simulink model "MIAC_ZTransform_PLC_Coder_not_external"  (R2018b)
settings: Solver=FixedStepDiscrete  StartTime=0.0  StopTime=20  FixedStep=1  RelTol=1e-3
libraries: simulink x2, slident x2
settings Model: Creator=Trips  LastModifiedBy=Trips
settings ConfigComp: PLC_OutputDir=PLCCoder  PLC_TargetIDE=step7  PLC_GenerateReport=off  PLC_LaunchReport=off

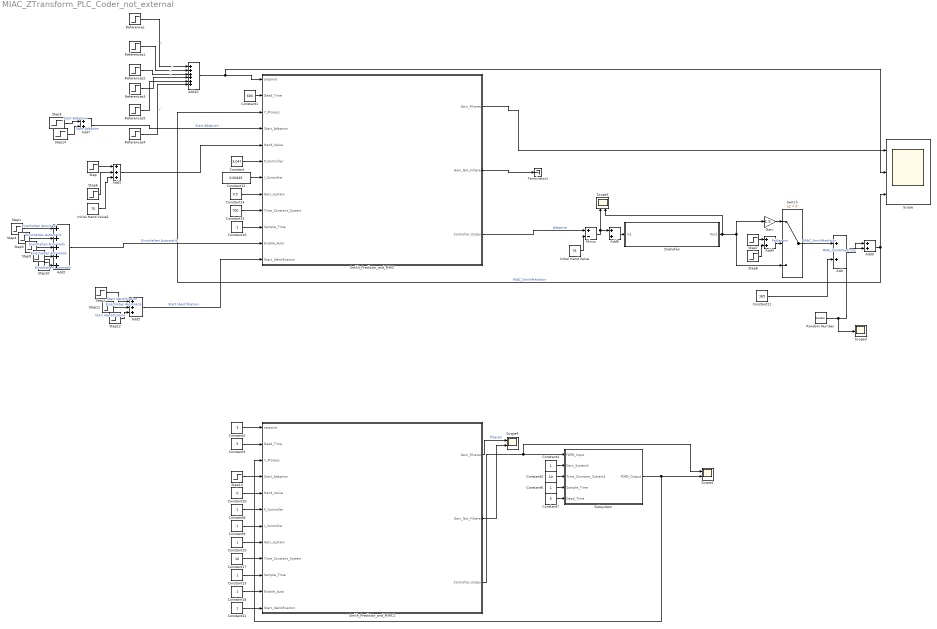
== system MIAC_ZTransform_PLC_Coder_not_external ==
  Add{,3..4,6..7} (5 alike) : Sum
  Add1 : Sum  Inputs=+++
  Add10 : Sum  Inputs=++++++
  Add2 : Sum  Inputs=5
  Add5 : Sum  Inputs=+++
  Constant : Constant  Value=3.047
  Constant1 : Constant  Value=600
  Constant{4,6,8..10,13,16,18,21} (9 alike) : Constant
  Constant11 : Constant  Value=165
  Constant12 : Constant  Value=0.00445
  Constant14 : Constant  Value=0.5
  Constant15 : Constant  Value=700
  Constant17 : Constant  Value=10
  Constant2 : Constant  Value=3
  Constant20 : Constant  Value=0
  Constant3 : Constant  Value=5
  Constant5 : Constant  Value=10
  Constant7 : Constant  Value=5
  Drehofen : Subsystem
  Gain : Gain  Gain=1.5
  Initial Hand Value : Constant  Value=75
  Initial Hand Value1 : Constant  Value=75
  Minus : Sum  Inputs=+-
  Random Number : RandomNumber  Variance=0.01  SampleTime=10
  References : Step  After=3
  References1 : Step  Time=12000  After=2
  References2 : Step  Time=18000  After=3
  References3 : Step  Time=35000  After=3
  References4 : Step  Time=0  After=165
  References5 : Step  Time=40000  After=-7
  Scope : Scope  NumInputPorts=3
  Scope1 : Scope  NumInputPorts=2
  Scope2 : Scope  NumInputPorts=2
  Scope3 : Scope
  Scope4 : Scope  NumInputPorts=2
  Smith_Predictor_and_MIAC : Subsystem  TreatAsAtomicUnit=on  SystemSampleTime=1
  Smith_Predictor_and_MIAC1 : Subsystem  TreatAsAtomicUnit=on  SystemSampleTime=1
  Step : Step  Time=300  After=5  SampleTime=0
  Step1 : Step  Time=4000  SampleTime=0
  Step10 : Step  Time=50000  SampleTime=0
  Step11 : Step  Time=35000  After=-1  SampleTime=0
  Step12 : Step  Time=38000  SampleTime=1
  Step13 : Step  Time=500  SampleTime=0
  Step14 : Step  Time=2.5*10^4  SampleTime=1
  Step2 : Step  Time=3900  SampleTime=1
  Step3 : Step  Time=5000  Before=1  After=0  SampleTime=1
  Step4 : Step  Time=20000  After=-1  SampleTime=0
  Step5 : Step  Time=25000  SampleTime=0
  Step6 : Step  Time=19000  After=5  SampleTime=0
  Step7 : Step  Time=3*10^4  SampleTime=0
  Step8 : Step  Time=3.8*10^4  After=0  SampleTime=0
  Step9 : Step  Time=45000  After=-1  SampleTime=0
  Subsystem : Subsystem  TreatAsAtomicUnit=on  SystemSampleTime=1
  Switch : Switch  Criteria=u2 > Threshold
  Terminator1 : Terminator
  wires:
  Smith_Predictor_and_MIAC/1(Gain_Filtered) -> Scope/1
  Smith_Predictor_and_MIAC/2(Gain_Not_Filtered) -> Terminator1/1
  Add10/1 -> Scope/2, Smith_Predictor_and_MIAC/1(setpoint)
  Step8/1 -> Add4/2
  Smith_Predictor_and_MIAC/3(Controller_Output) -> Minus/1  "Adaptive"
  Add4/1 -> Switch/2  "Fehler ein"
  Gain/1 -> Switch/1
  Minus/1 -> Add6/1, Scope1/1
  Add6/1 -> Drehofen/1(In1)
  Drehofen/1(Out1) -> Scope1/2, Gain/1, Switch/3
  Step7/1 -> Add4/1
  Random Number/1 -> Scope3/1, Add3/2
  Initial Hand Value/1 -> Minus/2
  Add/1 -> Add3/1  "MIAC_SmithPredictor"
  Switch/1 -> Add/1  "MIAC_SmithPredictor"
  Constant11/1 -> Add/2
  Add3/1 -> Scope/3, Smith_Predictor_and_MIAC/3(Y_Process)  "MIAC_SmithPredictor"
  References3/1 -> Add10/4  "r"
  References/1 -> Add10/1  "r"
  References4/1 -> Add10/6  "r"
  References1/1 -> Add10/2  "r"
  References2/1 -> Add10/3  "r"
  References5/1 -> Add10/5
  Constant/1 -> Smith_Predictor_and_MIAC/6(P_Controller)
  Constant12/1 -> Smith_Predictor_and_MIAC/7(I_Controller)
  Constant14/1 -> Smith_Predictor_and_MIAC/8(Gain_System)
  Constant15/1 -> Smith_Predictor_and_MIAC/9(Time_Constant_System)
  Constant16/1 -> Smith_Predictor_and_MIAC/10(Sample_Time)
  Constant1/1 -> Smith_Predictor_and_MIAC/2(Dead_Time)
  Step14/1 -> Add7/2  "Start Adaption"
  Step3/1 -> Add7/1  "Start Adaption"
  Add7/1 -> Smith_Predictor_and_MIAC/4(Start_Adaption)  "Start Adaption"
  Step6/1 -> Add1/2
  Initial Hand Value1/1 -> Add1/3
  Step/1 -> Add1/1
  Add1/1 -> Smith_Predictor_and_MIAC/5(Hand_Value)
  Step9/1 -> Add2/4  "Einschalten Automatik"
  Step10/1 -> Add2/5  "Einschalten Automatik"
  Step5/1 -> Add2/3  "Einschalten Automatik"
  Step4/1 -> Add2/2  "Einschalten Automatik"
  Step1/1 -> Add2/1  "Einschalten Automatik"
  Add2/1 -> Smith_Predictor_and_MIAC/11(" Enable_Auto")  "Einschalten Automatik"
  Step12/1 -> Add5/3  "Start Identification"
  Step11/1 -> Add5/2  "Einschalten Automatik"
  Step2/1 -> Add5/1  "Start Identification"
  Add5/1 -> Smith_Predictor_and_MIAC/12(Start_Identification)  "Start Identification"
  Constant2/1 -> Smith_Predictor_and_MIAC1/1(setpoint)
  Constant3/1 -> Smith_Predictor_and_MIAC1/2(Dead_Time)
  Constant7/1 -> Subsystem/5(" Dead_Time")
  Constant4/1 -> Subsystem/2(Gain_System1)
  Constant6/1 -> Subsystem/4(Sample_Time)
  Subsystem/1(FOPD_Output) -> Smith_Predictor_and_MIAC1/3(Y_Process), Scope2/2
  Constant5/1 -> Subsystem/3(Time_Constant_System1)
  Smith_Predictor_and_MIAC1/3(Controller_Output) -> Scope2/1, Subsystem/1(FOPD_Input)
  Constant8/1 -> Smith_Predictor_and_MIAC1/6(P_Controller)
  Constant9/1 -> Smith_Predictor_and_MIAC1/7(I_Controller)
  Constant10/1 -> Smith_Predictor_and_MIAC1/8(Gain_System)
  Constant13/1 -> Smith_Predictor_and_MIAC1/10(Sample_Time)
  Constant17/1 -> Smith_Predictor_and_MIAC1/9(Time_Constant_System)
  Constant18/1 -> Smith_Predictor_and_MIAC1/11(" Enable_Auto")
  Step13/1 -> Smith_Predictor_and_MIAC1/4(Start_Adaption)
  Constant20/1 -> Smith_Predictor_and_MIAC1/5(Hand_Value)
  Constant21/1 -> Smith_Predictor_and_MIAC1/12(Start_Identification)
  Smith_Predictor_and_MIAC1/1(Gain_Filtered) -> Scope4/1  "filtered"
  Smith_Predictor_and_MIAC1/2(Gain_Not_Filtered) -> Scope4/2

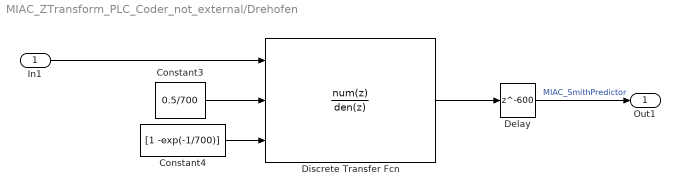
== system MIAC_ZTransform_PLC_Coder_not_external/Drehofen ==
  In1 : Inport
  Constant3 : Constant  Value=0.5/700
  Constant4 : Constant  Value=[1 -exp(-1/700)]
  Delay : Delay  DelayLength=600
  Discrete Transfer Fcn : DiscreteTransferFcn  NumeratorSource=Input port  DenominatorSource=Input port  a0EqualsOne=on
      settings: InputPortMap=u0,p1,p3
  Out1 : Outport
  wires:
  Discrete Transfer Fcn/1 -> Delay/1
  Constant4/1 -> Discrete Transfer Fcn/3
  Constant3/1 -> Discrete Transfer Fcn/2
  In1/1 -> Discrete Transfer Fcn/1
  Delay/1 -> Out1/1  "MIAC_SmithPredictor"

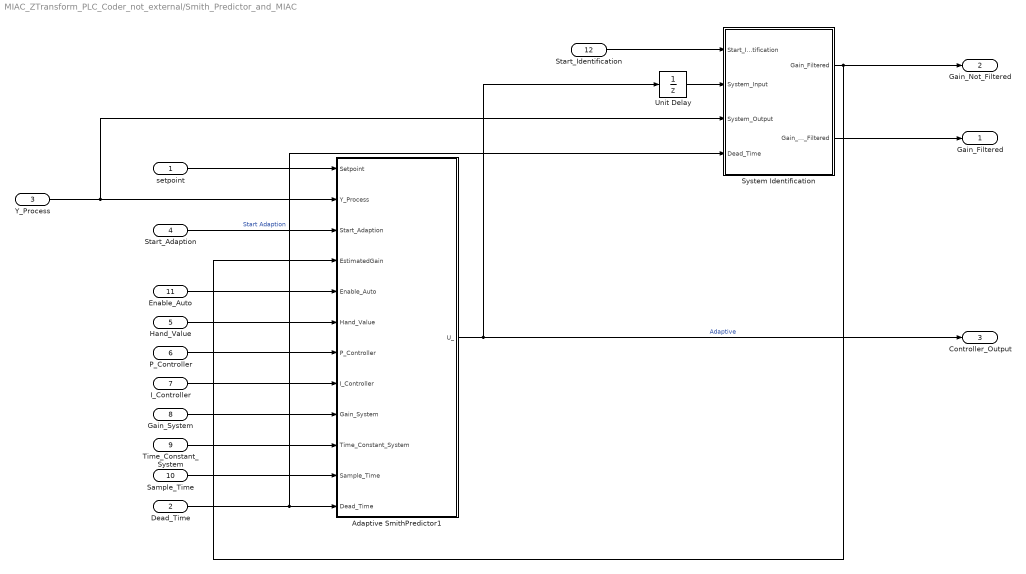
== system MIAC_ZTransform_PLC_Coder_not_external/Smith_Predictor_and_MIAC ==
  setpoint : Inport
  Dead_Time : Inport  Port=2
  Y_Process : Inport  Port=3
  Start_Adaption : Inport  Port=4
  Hand_Value : Inport  Port=5
  P_Controller : Inport  Port=6
  I_Controller : Inport  Port=7
  Gain_System : Inport  Port=8
  Time_Constant_System : Inport  Port=9
  Sample_Time : Inport  Port=10
  " Enable_Auto" : Inport  Port=11
  Start_Identification : Inport  Port=12  PortDimensions=1  SampleTime=1
  Adaptive SmithPredictor1 : Subsystem  TreatAsAtomicUnit=on  SystemSampleTime=1
  System Identification : Subsystem  TreatAsAtomicUnit=on  SystemSampleTime=1
  Unit Delay : UnitDelay  SampleTime=-1
  Gain_Filtered : Outport
  Gain_Not_Filtered : Outport  Port=2
  Controller_Output : Outport  Port=3
  wires:
  Gain_System/1 -> Adaptive SmithPredictor1/9(Gain_System)
  Dead_Time/1 -> Adaptive SmithPredictor1/12(" Dead_Time"), System Identification/4(Dead_Time)
  Adaptive SmithPredictor1/1(U_) -> Unit Delay/1, Controller_Output/1  "Adaptive"
  Time_Constant_System/1 -> Adaptive SmithPredictor1/10(Time_Constant_System)
  P_Controller/1 -> Adaptive SmithPredictor1/7(P_Controller)
  Sample_Time/1 -> Adaptive SmithPredictor1/11(Sample_Time)
  I_Controller/1 -> Adaptive SmithPredictor1/8(I_Controller)
  Start_Adaption/1 -> Adaptive SmithPredictor1/3(Start_Adaption)  "Start Adaption"
  System Identification/2(Gain_Not_Filtered) -> Gain_Filtered/1
  setpoint/1 -> Adaptive SmithPredictor1/1(Setpoint)
  Start_Identification/1 -> System Identification/1(Start_Identification)
  System Identification/1(Gain_Filtered) -> Adaptive SmithPredictor1/4(EstimatedGain), Gain_Not_Filtered/1
  " Enable_Auto"/1 -> Adaptive SmithPredictor1/5(Enable_Auto)
  Hand_Value/1 -> Adaptive SmithPredictor1/6(Hand_Value)
  Y_Process/1 -> System Identification/3(System_Output), Adaptive SmithPredictor1/2(Y_Process)
  Unit Delay/1 -> System Identification/2(System_Input)

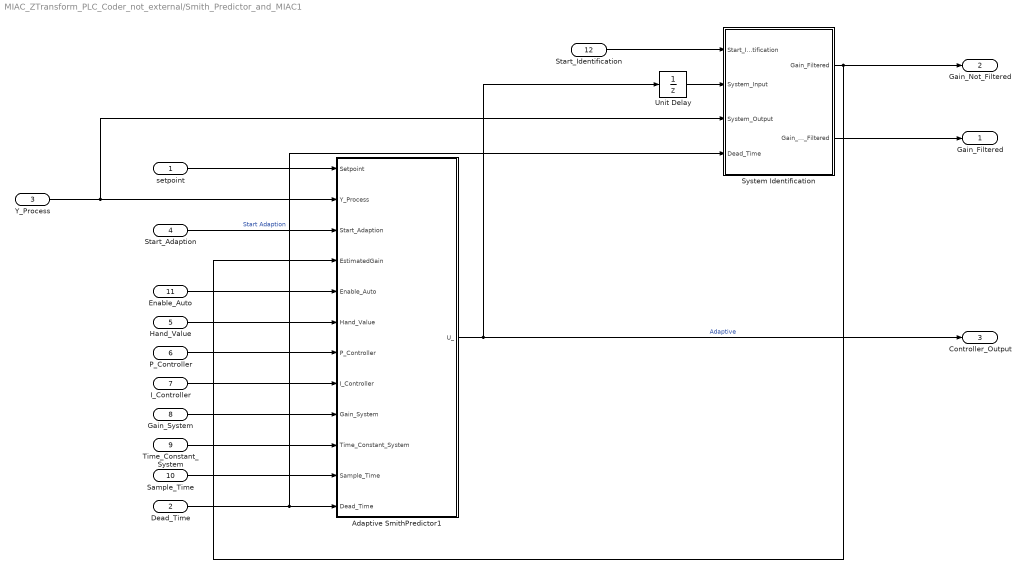
== system MIAC_ZTransform_PLC_Coder_not_external/Smith_Predictor_and_MIAC1 ==
  setpoint : Inport
  Dead_Time : Inport  Port=2
  Y_Process : Inport  Port=3
  Start_Adaption : Inport  Port=4
  Hand_Value : Inport  Port=5
  P_Controller : Inport  Port=6
  I_Controller : Inport  Port=7
  Gain_System : Inport  Port=8
  Time_Constant_System : Inport  Port=9
  Sample_Time : Inport  Port=10
  " Enable_Auto" : Inport  Port=11
  Start_Identification : Inport  Port=12  PortDimensions=1  SampleTime=1
  Adaptive SmithPredictor1 : Subsystem  TreatAsAtomicUnit=on  SystemSampleTime=1
  System Identification : Subsystem  TreatAsAtomicUnit=on  SystemSampleTime=1
  Unit Delay : UnitDelay  SampleTime=-1
  Gain_Filtered : Outport
  Gain_Not_Filtered : Outport  Port=2
  Controller_Output : Outport  Port=3
  wires:
  Gain_System/1 -> Adaptive SmithPredictor1/9(Gain_System)
  Dead_Time/1 -> Adaptive SmithPredictor1/12(" Dead_Time"), System Identification/4(Dead_Time)
  Adaptive SmithPredictor1/1(U_) -> Unit Delay/1, Controller_Output/1  "Adaptive"
  Time_Constant_System/1 -> Adaptive SmithPredictor1/10(Time_Constant_System)
  P_Controller/1 -> Adaptive SmithPredictor1/7(P_Controller)
  Sample_Time/1 -> Adaptive SmithPredictor1/11(Sample_Time)
  I_Controller/1 -> Adaptive SmithPredictor1/8(I_Controller)
  Start_Adaption/1 -> Adaptive SmithPredictor1/3(Start_Adaption)  "Start Adaption"
  System Identification/2(Gain_Not_Filtered) -> Gain_Filtered/1
  setpoint/1 -> Adaptive SmithPredictor1/1(Setpoint)
  Start_Identification/1 -> System Identification/1(Start_Identification)
  System Identification/1(Gain_Filtered) -> Adaptive SmithPredictor1/4(EstimatedGain), Gain_Not_Filtered/1
  " Enable_Auto"/1 -> Adaptive SmithPredictor1/5(Enable_Auto)
  Hand_Value/1 -> Adaptive SmithPredictor1/6(Hand_Value)
  Y_Process/1 -> System Identification/3(System_Output), Adaptive SmithPredictor1/2(Y_Process)
  Unit Delay/1 -> System Identification/2(System_Input)

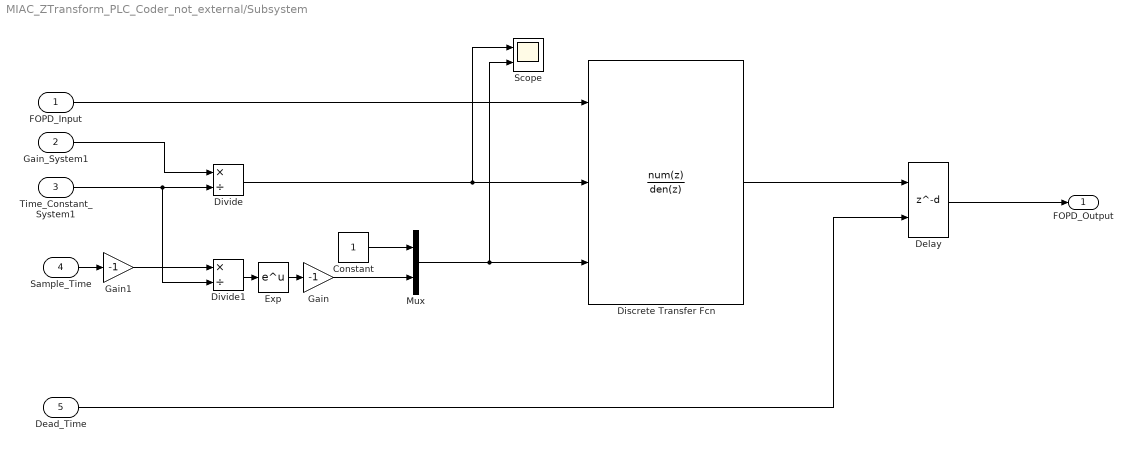
== system MIAC_ZTransform_PLC_Coder_not_external/Subsystem ==
  FOPD_Input : Inport
  Gain_System1 : Inport  Port=2
  Time_Constant_System1 : Inport  Port=3
  Sample_Time : Inport  Port=4
  " Dead_Time" : Inport  Port=5
  Constant : Constant
  Delay : Delay  DelayLengthSource=Input port  DelayLength=600  DelayLengthUpperLimit=800
      settings: InputPortMap=u0,p1
  Discrete Transfer Fcn : DiscreteTransferFcn  NumeratorSource=Input port  DenominatorSource=Input port  a0EqualsOne=on
      settings: InputPortMap=u0,p1,p3
  Divide : Product  Inputs=*/
  Divide1 : Product  Inputs=*/
  Exp : Math  SaturateOnIntegerOverflow=on
  Gain : Gain  Gain=-1
  Gain1 : Gain  Gain=-1
  Mux : Mux  Inputs=2
  Scope : Scope  NumInputPorts=2
  FOPD_Output : Outport
  wires:
  Gain1/1 -> Divide1/1
  Time_Constant_System1/1 -> Divide1/2, Divide/2
  FOPD_Input/1 -> Discrete Transfer Fcn/1
  Discrete Transfer Fcn/1 -> Delay/1
  Exp/1 -> Gain/1
  Constant/1 -> Mux/1
  Mux/1 -> Scope/2, Discrete Transfer Fcn/3
  Divide1/1 -> Exp/1
  Gain_System1/1 -> Divide/1
  Gain/1 -> Mux/2
  " Dead_Time"/1 -> Delay/2
  Sample_Time/1 -> Gain1/1
  Divide/1 -> Scope/1, Discrete Transfer Fcn/2
  Delay/1 -> FOPD_Output/1

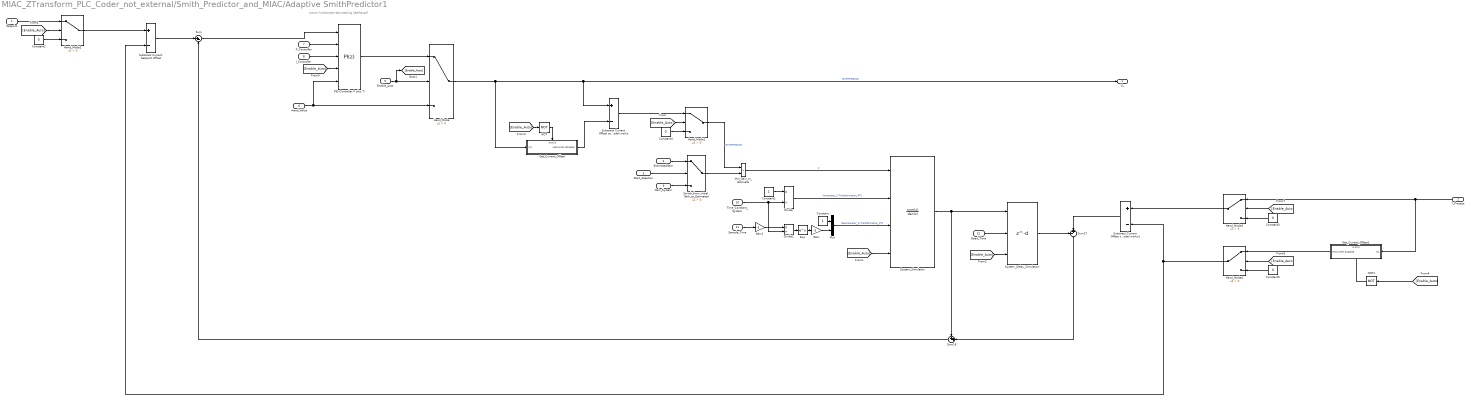
== system MIAC_ZTransform_PLC_Coder_not_external/Smith_Predictor_and_MIAC/Adaptive SmithPredictor1 ==
  note: warum funktioniert das tracking überhaupt?
  Setpoint : Inport
  Y_Process : Inport  Port=2
  Start_Adaption : Inport  Port=3
  EstimatedGain : Inport  Port=4
  Enable_Auto : Inport  Port=5
  Hand_Value : Inport  Port=6
  P_Controller : Inport  Port=7
  I_Controller : Inport  Port=8
  Gain_System : Inport  Port=9
  Time_Constant_System : Inport  Port=10
  Sample_Time : Inport  Port=11
  " Dead_Time" : Inport  Port=12
  Constant : Constant
  Constant1 : Constant
  Constant{2..5} (4 alike) : Constant  Value=0
  Divide : Product  Inputs=*/
  Divide1 : Product  Inputs=*/
  Exp : Math  SaturateOnIntegerOverflow=on
  Gain : Gain  Gain=-1
  Gain1 : Gain  Gain=-1
  Get_Current_Offset : Subsystem
  Get_Current_Offset1 : Subsystem
  Hand_Mode{,1..4} (5 alike) : Switch  Criteria=u2 > Threshold
  Mul_Gain_or_Estimate : Product
  Mux : Mux  Inputs=2
  NOT : Logic  Operator=NOT  IconShape=distinctive  AllPortsSameDT=off  OutDataTypeStr=boolean
  NOT1 : Logic  Operator=NOT  IconShape=distinctive  AllPortsSameDT=off  OutDataTypeStr=boolean
  "PID Controller P plus Ti " : simulink/Continuous/PID Controller  Controller=PI  Form=Parallel  TimeDomain=Discrete-time  SampleTime=1  IntegratorMethod=Forward Euler  FilterMethod=Forward Euler  ControllerParametersSource=external  P=3.04732259067536  I=0.00445689106465138  D=118.272348286844  UseFilter=on  N=0.00420306193364532  TunerSelectOption=Transfer Function Based (PID Tuner App)  InitialConditionSource=external  InitialConditionForIntegrator=0  InitialConditionForFilter=0  DifferentiatorICPrevScaledInput=0  ExternalReset=rising  TrackingMode=off  Kt=1  LimitOutput=on  UpperSaturationLimit=100  LowerSaturationLimit=0  LinearizeAsGain=on  AntiWindupMode=none  Kb=1  POutMin=[]  POutMax=[]  IOutMin=[]  IOutMax=[]  DOutMin=[]  DOutMax=[]  NOutMin=[]  NOutMax=[]  SumOutMin=[]  SumOutMax=[]  SaturationOutMin=[]  SaturationOutMax=[]  PParamMin=[]  PParamMax=[]  IParamMin=[]  IParamMax=[]  DParamMin=[]  DParamMax=[]  NParamMin=[]  NParamMax=[]  KbParamMin=[]  KbParamMax=[]  KtParamMin=[]  KtParamMax=[]  KbOutMin=[]  KbOutMax=[]  KtOutMin=[]  KtOutMax=[]  IntegratorOutMin=[]  IntegratorOutMax=[]  FilterOutMin=[]  FilterOutMax=[]  SumI1OutMin=[]  SumI1OutMax=[]  SumI2OutMin=[]  SumI2OutMax=[]  SumI3OutMin=[]  SumI3OutMax=[]  SumI4OutMin=[]  SumI4OutMax=[]  SumDOutMin=[]  SumDOutMax=[]  DifferentiatorOutMin=[]  DifferentiatorOutMax=[]  FilterDiffOutCoefMin=[]  FilterDiffOutCoefMax=[]  ReciprocalOutMin=[]  ReciprocalOutMax=[]  SumDenOutMin=[]  SumDenOutMax=[]  SumNumOutMin=[]  SumNumOutMax=[]  DivideOutMin=[]  DivideOutMax=[]  IntegratorContinuousStateAttributes=''  IntegratorStateMustResolveToSignalObject=off  IntegratorRTWStateStorageClass=Auto  FilterContinuousStateAttributes=''  FilterStateMustResolveToSignalObject=off  FilterRTWStateStorageClass=Auto  ParallelPVariant=ExternalParameters  IdealPVariant=Disabled  IVariant=ExternalParameters  DVariant=Disabled  IntegratorVariant=Discrete  SatVariant=Enabled  AWVariant=Passthrough  PCopyVariant=Disabled  TRVariant=Disabled  FdbkBlocksVariant=Forward  IdealPFdbkVariant=Disabled  SatFdbkVariant=Disabled  DerivativeFilterVariant=Disabled  NVariant=Disabled  NCopyVariant=Disabled_SignalSpec  FilterICVariant=Disabled  IntegratorICVariant=ExternalICs  ExternalResetVariant=ExternalReset  TRSumVariant=Passthrough  SumFdbkVariant=Disabled  SumVariant=Sum_PI
  Substract Current Offset so that the linearised model works : Sum  Inputs=+-
  Substract Current Offset so that the linearised model works1 : Sum  Inputs=+-
  Substract Current Setpoint Offset : Sum  Inputs=+-
  Sum : Sum  Inputs=|+-
  Sum17 : Sum  Inputs=-+|
  Sum18 : Sum  Inputs=++|
  Switch_from_initial_Gain_to_Estimated : Switch  Criteria=u2 > Threshold
  System_Delay_Simulation : Delay  DelayLengthSource=Input port  DelayLength=600  DelayLengthUpperLimit=800  ExternalReset=Rising  SampleTime=1
      settings: InputPortMap=u0,p1,r5
  System_Simulaton : DiscreteTransferFcn  NumeratorSource=Input port  DenominatorSource=Input port  ExternalReset=Rising  SampleTime=1  a0EqualsOne=on
      settings: InputPortMap=u0,p1,p3,r7
  U_ : Outport
  wires:
  Substract Current Setpoint Offset/1 -> Sum/1
  Sum/1 -> "PID Controller P plus Ti "/1
  Hand_Mode/1 -> U_/1, Substract Current Offset so that the linearised model works/1, Get_Current_Offset/1(In1)  "SmithPredictor"
  Substract Current Offset so that the linearised model works1/1 -> Sum17/2
  System_Simulaton/1 -> Sum18/1, System_Delay_Simulation/1
  System_Delay_Simulation/1 -> Sum17/1
  Sum17/1 -> Sum18/2
  Mul_Gain_or_Estimate/1 -> System_Simulaton/1  "U"
  Switch_from_initial_Gain_to_Estimated/1 -> Mul_Gain_or_Estimate/2
  "PID Controller P plus Ti "/1 -> Hand_Mode/1
  Hand_Value/1 -> "PID Controller P plus Ti "/5, Hand_Mode/3
  Enable_Auto/1 -> [Enable_Auto], Hand_Mode/2
  P_Controller/1 -> "PID Controller P plus Ti "/2
  I_Controller/1 -> "PID Controller P plus Ti "/3
  Divide/1 -> System_Simulaton/2  "Numerator_Z-Transformation_PT1"
  Mux/1 -> System_Simulaton/3  "Denumerator_Z-Transformation_PT1"
  Time_Constant_System/1 -> Divide1/2, Divide/2
  Constant/1 -> Mux/1
  Exp/1 -> Gain/1
  Gain/1 -> Mux/2
  Divide1/1 -> Exp/1
  Sample_Time/1 -> Gain1/1
  " Dead_Time"/1 -> System_Delay_Simulation/2
  Gain_System/1 -> Switch_from_initial_Gain_to_Estimated/3
  Start_Adaption/1 -> Switch_from_initial_Gain_to_Estimated/2
  EstimatedGain/1 -> Switch_from_initial_Gain_to_Estimated/1
  Constant1/1 -> Divide/1
  Gain1/1 -> Divide1/1
  [Enable_Auto] -> Hand_Mode1/2
  Hand_Mode1/1 -> Mul_Gain_or_Estimate/1  "SmithPredictor"
  Constant4/1 -> Hand_Mode1/3
  [Enable_Auto] -> System_Simulaton/4
  [Enable_Auto] -> System_Delay_Simulation/3
  Substract Current Offset so that the linearised model works/1 -> Hand_Mode1/1
  Get_Current_Offset/1(Hold when disabled) -> Substract Current Offset so that the linearised model works/2
  [Enable_Auto] -> NOT/1
  NOT/1 -> Get_Current_Offset/Enable
  Sum18/1 -> Sum/2
  Hand_Mode2/1 -> Substract Current Setpoint Offset/1
  NOT1/1 -> Get_Current_Offset1/Enable
  [Enable_Auto] -> NOT1/1
  Hand_Mode4/1 -> Substract Current Setpoint Offset/2, Substract Current Offset so that the linearised model works1/2
  [Enable_Auto] -> "PID Controller P plus Ti "/4
  Setpoint/1 -> Hand_Mode2/1
  [Enable_Auto] -> Hand_Mode2/2
  Constant2/1 -> Hand_Mode2/3
  Y_Process/1 -> Get_Current_Offset1/1(In1), Hand_Mode3/1
  [Enable_Auto] -> Hand_Mode3/2
  Constant3/1 -> Hand_Mode3/3
  Hand_Mode3/1 -> Substract Current Offset so that the linearised model works1/1
  Constant5/1 -> Hand_Mode4/3
  [Enable_Auto] -> Hand_Mode4/2
  Get_Current_Offset1/1(Hold when disabled) -> Hand_Mode4/1

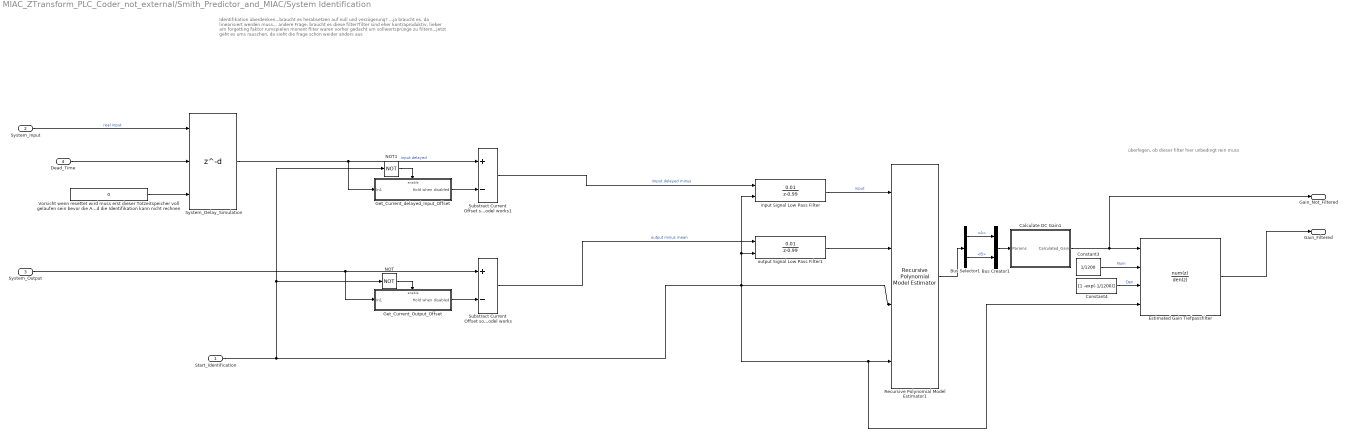
== system MIAC_ZTransform_PLC_Coder_not_external/Smith_Predictor_and_MIAC/System Identification ==
  note: überlegen, ob dieser filter hier unbedingt rein muss
  note: Identifikation überdenken...braucht es herabsetzen auf null und verzögerung?
      | ...ja braucht es, da linearisiert werden muss...
      |
      | andere Frage, braucht es diese filter?filter sind eher kontraproduktiv, lieber am forgetting faktor rumspielen
      | monent fliter waren vorher gedacht um sollwertsprünge zu filtern...jetzt geht es ums rauschen, da sieht die frage schon weider anders aus
  Start_Identification : Inport  SampleTime=1
  System_Input : Inport  Port=2
  System_Output : Inport  Port=3  SampleTime=1
  Dead_Time : Inport  Port=4
  Bus Creator1 : BusCreator  Inputs=2
  Bus Selector1 : BusSelector  OutputSignals=A,B
  Calculate DC Gain1 : Subsystem  TreatAsAtomicUnit=on  SystemSampleTime=1
  Constant3 : Constant  Value=1/1200
  Constant4 : Constant  Value=[1 -exp(-1/1200)]
  Estimated Gain Tiefpassfilter : DiscreteTransferFcn  NumeratorSource=Input port  DenominatorSource=Input port  ExternalReset=Rising  a0EqualsOne=on
      settings: InputPortMap=u0,p1,p3,r7
  Get_Current_Output_Offset : Subsystem
  Get_Current_delayed_Input_Offset : Subsystem
  NOT : Logic  Operator=NOT  IconShape=distinctive  AllPortsSameDT=off  OutDataTypeStr=boolean
  NOT1 : Logic  Operator=NOT  IconShape=distinctive  AllPortsSameDT=off  OutDataTypeStr=boolean
  Recursive Polynomial Model Estimator1 : slident/Estimators/Recursive Polynomial Model Estimator  ModelStructure=ARX  InitialEstimateSource=None  A0=2  B0=1  C0=1  D0=1  F0=1  nk=1  P0=10  InitialInputs=0  InitialOutputs=0  History=Infinite  WindowLength=2000  EstimationMethod=Forgetting Factor  AdaptationParameter=1  HasTimeVaryingAdaptationParameter=off  NormalizationBias=eps  OutputError=off  OutputP=off  AddEnablePort=on  ExternalReset=Rising  InputProcessing=Sample-based  Ts=1
      settings: SourceProductName=System Identification Toolbox  SourceProductBaseCode=ID
  Substract Current Offset so that the linearised model works : Sum  Inputs=+-
  Substract Current Offset so that the linearised model works1 : Sum  Inputs=+-
  System_Delay_Simulation : Delay  DelayLengthSource=Input port  DelayLength=600  DelayLengthUpperLimit=800  ExternalReset=Rising  SampleTime=1
      settings: InputPortMap=u0,p1,r5
  Vorsicht wenn resettet wird muss erst dieser Totzeitspeicher voll gelaufen sein bevor die Adaption starten darf Sonst kommt heir immer 0 raus und die Identifikation kann nicht rechnen : Constant  Value=0
  input Signal Low Pass Filter : DiscreteTransferFcn  Numerator=[0.01]  Denominator=[1 -0.99]  ExternalReset=Rising  SampleTime=1  a0EqualsOne=on
      settings: InputPortMap=u0,r7
  output Signal Low Pass Filter1 : DiscreteTransferFcn  Numerator=[0.01]  Denominator=[1 -0.99]  ExternalReset=Rising  SampleTime=1  a0EqualsOne=on
      settings: InputPortMap=u0,r7
  Gain_Filtered : Outport
  Gain_Not_Filtered : Outport  Port=2
  wires:
  Recursive Polynomial Model Estimator1/1 -> Bus Selector1/1
  input Signal Low Pass Filter/1 -> Recursive Polynomial Model Estimator1/1  "input"
  Bus Creator1/1 -> Calculate DC Gain1/1(Params)
  Bus Selector1/1 -> Bus Creator1/1  "<A>"
  Bus Selector1/2 -> Bus Creator1/2  "<B>"
  Substract Current Offset so that the linearised model works/1 -> output Signal Low Pass Filter1/1  "output minus mean"
  NOT/1 -> Get_Current_Output_Offset/Enable
  Get_Current_Output_Offset/1(Hold when disabled) -> Substract Current Offset so that the linearised model works/2
  System_Output/1 -> Get_Current_Output_Offset/1(In1), Substract Current Offset so that the linearised model works/1
  Get_Current_delayed_Input_Offset/1(Hold when disabled) -> Substract Current Offset so that the linearised model works1/2
  NOT1/1 -> Get_Current_delayed_Input_Offset/Enable
  Estimated Gain Tiefpassfilter/1 -> Gain_Filtered/1
  System_Input/1 -> System_Delay_Simulation/1  "real input"
  Vorsicht wenn resettet wird muss erst dieser Totzeitspeicher voll gelaufen sein bevor die Adaption starten darf Sonst kommt heir immer 0 raus und die Identifikation kann nicht rechnen/1 -> System_Delay_Simulation/3
  Dead_Time/1 -> System_Delay_Simulation/2
  Substract Current Offset so that the linearised model works1/1 -> input Signal Low Pass Filter/1  "imput delayed minus"
  System_Delay_Simulation/1 -> Substract Current Offset so that the linearised model works1/1, Get_Current_delayed_Input_Offset/1(In1)  "input delayed"
  Calculate DC Gain1/1(Calculated_Gain) -> Gain_Not_Filtered/1, Estimated Gain Tiefpassfilter/1
  Constant3/1 -> Estimated Gain Tiefpassfilter/2  "Num"
  Constant4/1 -> Estimated Gain Tiefpassfilter/3  "Den"
  Start_Identification/1 -> NOT/1, NOT1/1, Estimated Gain Tiefpassfilter/4, Recursive Polynomial Model Estimator1/4, output Signal Low Pass Filter1/2, input Signal Low Pass Filter/2, Recursive Polynomial Model Estimator1/3
  output Signal Low Pass Filter1/1 -> Recursive Polynomial Model Estimator1/2

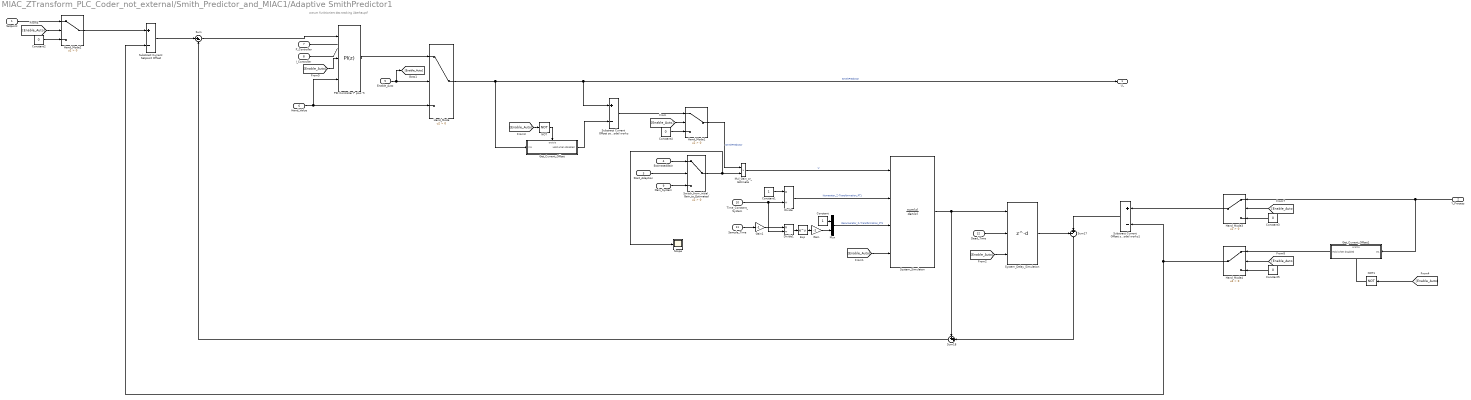
== system MIAC_ZTransform_PLC_Coder_not_external/Smith_Predictor_and_MIAC1/Adaptive SmithPredictor1 ==
  note: warum funktioniert das tracking überhaupt?
  Setpoint : Inport
  Y_Process : Inport  Port=2
  Start_Adaption : Inport  Port=3
  EstimatedGain : Inport  Port=4
  Enable_Auto : Inport  Port=5
  Hand_Value : Inport  Port=6
  P_Controller : Inport  Port=7
  I_Controller : Inport  Port=8
  Gain_System : Inport  Port=9
  Time_Constant_System : Inport  Port=10
  Sample_Time : Inport  Port=11
  " Dead_Time" : Inport  Port=12
  Constant : Constant
  Constant1 : Constant
  Constant{2..5} (4 alike) : Constant  Value=0
  Divide : Product  Inputs=*/
  Divide1 : Product  Inputs=*/
  Exp : Math  SaturateOnIntegerOverflow=on
  Gain : Gain  Gain=-1
  Gain1 : Gain  Gain=-1
  Get_Current_Offset : Subsystem
  Get_Current_Offset1 : Subsystem
  Hand_Mode{,1..4} (5 alike) : Switch  Criteria=u2 > Threshold
  Mul_Gain_or_Estimate : Product
  Mux : Mux  Inputs=2
  NOT : Logic  Operator=NOT  IconShape=distinctive  AllPortsSameDT=off  OutDataTypeStr=boolean
  NOT1 : Logic  Operator=NOT  IconShape=distinctive  AllPortsSameDT=off  OutDataTypeStr=boolean
  "PID Controller P plus Ti " : simulink/Continuous/PID Controller  Controller=PI  Form=Parallel  TimeDomain=Discrete-time  SampleTime=1  IntegratorMethod=Forward Euler  FilterMethod=Forward Euler  ControllerParametersSource=internal  P=2.6486842094067  I=0.282118907823572  D=118.272348286844  UseFilter=on  N=0.00420306193364532  TunerSelectOption=Transfer Function Based (PID Tuner App)  InitialConditionSource=external  InitialConditionForIntegrator=0  InitialConditionForFilter=0  DifferentiatorICPrevScaledInput=0  ExternalReset=rising  TrackingMode=off  Kt=1  LimitOutput=on  UpperSaturationLimit=100  LowerSaturationLimit=0  LinearizeAsGain=on  AntiWindupMode=none  Kb=1  POutMin=[]  POutMax=[]  IOutMin=[]  IOutMax=[]  DOutMin=[]  DOutMax=[]  NOutMin=[]  NOutMax=[]  SumOutMin=[]  SumOutMax=[]  SaturationOutMin=[]  SaturationOutMax=[]  PParamMin=[]  PParamMax=[]  IParamMin=[]  IParamMax=[]  DParamMin=[]  DParamMax=[]  NParamMin=[]  NParamMax=[]  KbParamMin=[]  KbParamMax=[]  KtParamMin=[]  KtParamMax=[]  KbOutMin=[]  KbOutMax=[]  KtOutMin=[]  KtOutMax=[]  IntegratorOutMin=[]  IntegratorOutMax=[]  FilterOutMin=[]  FilterOutMax=[]  SumI1OutMin=[]  SumI1OutMax=[]  SumI2OutMin=[]  SumI2OutMax=[]  SumI3OutMin=[]  SumI3OutMax=[]  SumI4OutMin=[]  SumI4OutMax=[]  SumDOutMin=[]  SumDOutMax=[]  DifferentiatorOutMin=[]  DifferentiatorOutMax=[]  FilterDiffOutCoefMin=[]  FilterDiffOutCoefMax=[]  ReciprocalOutMin=[]  ReciprocalOutMax=[]  SumDenOutMin=[]  SumDenOutMax=[]  SumNumOutMin=[]  SumNumOutMax=[]  DivideOutMin=[]  DivideOutMax=[]  IntegratorContinuousStateAttributes=''  IntegratorStateMustResolveToSignalObject=off  IntegratorRTWStateStorageClass=Auto  FilterContinuousStateAttributes=''  FilterStateMustResolveToSignalObject=off  FilterRTWStateStorageClass=Auto  ParallelPVariant=InternalParameters  IdealPVariant=Disabled  IVariant=InternalParameters  DVariant=Disabled  IntegratorVariant=Discrete  SatVariant=Enabled  AWVariant=Passthrough  PCopyVariant=Disabled  TRVariant=Disabled  FdbkBlocksVariant=Forward  IdealPFdbkVariant=Disabled  SatFdbkVariant=Disabled  DerivativeFilterVariant=Disabled  NVariant=Disabled  NCopyVariant=Disabled_SignalSpec  FilterICVariant=Disabled  IntegratorICVariant=ExternalICs  ExternalResetVariant=ExternalReset  TRSumVariant=Passthrough  SumFdbkVariant=Disabled  SumVariant=Sum_PI
  Scope : Scope
  Substract Current Offset so that the linearised model works : Sum  Inputs=+-
  Substract Current Offset so that the linearised model works1 : Sum  Inputs=+-
  Substract Current Setpoint Offset : Sum  Inputs=+-
  Sum : Sum  Inputs=|+-
  Sum17 : Sum  Inputs=-+|
  Sum18 : Sum  Inputs=++|
  Switch_from_initial_Gain_to_Estimated : Switch  Criteria=u2 > Threshold
  System_Delay_Simulation : Delay  DelayLengthSource=Input port  DelayLength=600  DelayLengthUpperLimit=800  ExternalReset=Rising  SampleTime=1
      settings: InputPortMap=u0,p1,r5
  System_Simulaton : DiscreteTransferFcn  NumeratorSource=Input port  DenominatorSource=Input port  ExternalReset=Rising  SampleTime=1  a0EqualsOne=on
      settings: InputPortMap=u0,p1,p3,r7
  U_ : Outport
  wires:
  Substract Current Setpoint Offset/1 -> Sum/1
  Sum/1 -> "PID Controller P plus Ti "/1
  Hand_Mode/1 -> U_/1, Substract Current Offset so that the linearised model works/1, Get_Current_Offset/1(In1)  "SmithPredictor"
  Substract Current Offset so that the linearised model works1/1 -> Sum17/2
  System_Simulaton/1 -> Sum18/1, System_Delay_Simulation/1
  System_Delay_Simulation/1 -> Sum17/1
  Sum17/1 -> Sum18/2
  Mul_Gain_or_Estimate/1 -> System_Simulaton/1  "U"
  Switch_from_initial_Gain_to_Estimated/1 -> Scope/1, Mul_Gain_or_Estimate/2
  "PID Controller P plus Ti "/1 -> Hand_Mode/1
  Hand_Value/1 -> "PID Controller P plus Ti "/3, Hand_Mode/3
  Enable_Auto/1 -> [Enable_Auto], Hand_Mode/2
  P_Controller/1 -> ?
  I_Controller/1 -> ?
  Divide/1 -> System_Simulaton/2  "Numerator_Z-Transformation_PT1"
  Mux/1 -> System_Simulaton/3  "Denumerator_Z-Transformation_PT1"
  Time_Constant_System/1 -> Divide1/2, Divide/2
  Constant/1 -> Mux/1
  Exp/1 -> Gain/1
  Gain/1 -> Mux/2
  Divide1/1 -> Exp/1
  Sample_Time/1 -> Gain1/1
  " Dead_Time"/1 -> System_Delay_Simulation/2
  Gain_System/1 -> Switch_from_initial_Gain_to_Estimated/3
  Start_Adaption/1 -> Switch_from_initial_Gain_to_Estimated/2
  EstimatedGain/1 -> Switch_from_initial_Gain_to_Estimated/1
  Constant1/1 -> Divide/1
  Gain1/1 -> Divide1/1
  [Enable_Auto] -> Hand_Mode1/2
  Hand_Mode1/1 -> Mul_Gain_or_Estimate/1  "SmithPredictor"
  Constant4/1 -> Hand_Mode1/3
  [Enable_Auto] -> System_Simulaton/4
  [Enable_Auto] -> System_Delay_Simulation/3
  Substract Current Offset so that the linearised model works/1 -> Hand_Mode1/1
  Get_Current_Offset/1(Hold when disabled) -> Substract Current Offset so that the linearised model works/2
  [Enable_Auto] -> NOT/1
  NOT/1 -> Get_Current_Offset/Enable
  Sum18/1 -> Sum/2
  Hand_Mode2/1 -> Substract Current Setpoint Offset/1
  NOT1/1 -> Get_Current_Offset1/Enable
  [Enable_Auto] -> NOT1/1
  Hand_Mode4/1 -> Substract Current Setpoint Offset/2, Substract Current Offset so that the linearised model works1/2
  [Enable_Auto] -> "PID Controller P plus Ti "/2
  Setpoint/1 -> Hand_Mode2/1
  [Enable_Auto] -> Hand_Mode2/2
  Constant2/1 -> Hand_Mode2/3
  Y_Process/1 -> Get_Current_Offset1/1(In1), Hand_Mode3/1
  [Enable_Auto] -> Hand_Mode3/2
  Constant3/1 -> Hand_Mode3/3
  Hand_Mode3/1 -> Substract Current Offset so that the linearised model works1/1
  Constant5/1 -> Hand_Mode4/3
  [Enable_Auto] -> Hand_Mode4/2
  Get_Current_Offset1/1(Hold when disabled) -> Hand_Mode4/1

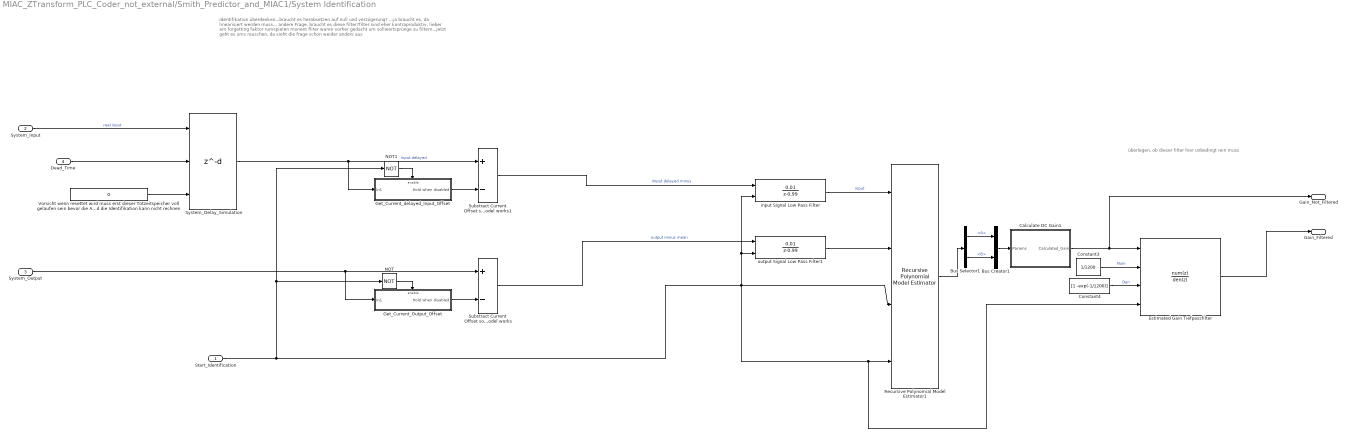
== system MIAC_ZTransform_PLC_Coder_not_external/Smith_Predictor_and_MIAC1/System Identification ==
  note: überlegen, ob dieser filter hier unbedingt rein muss
  note: Identifikation überdenken...braucht es herabsetzen auf null und verzögerung?
      | ...ja braucht es, da linearisiert werden muss...
      |
      | andere Frage, braucht es diese filter?filter sind eher kontraproduktiv, lieber am forgetting faktor rumspielen
      | monent fliter waren vorher gedacht um sollwertsprünge zu filtern...jetzt geht es ums rauschen, da sieht die frage schon weider anders aus
  Start_Identification : Inport  SampleTime=1
  System_Input : Inport  Port=2
  System_Output : Inport  Port=3  SampleTime=1
  Dead_Time : Inport  Port=4
  Bus Creator1 : BusCreator  Inputs=2
  Bus Selector1 : BusSelector  OutputSignals=A,B
  Calculate DC Gain1 : Subsystem  TreatAsAtomicUnit=on  SystemSampleTime=1
  Constant3 : Constant  Value=1/1200
  Constant4 : Constant  Value=[1 -exp(-1/1200)]
  Estimated Gain Tiefpassfilter : DiscreteTransferFcn  NumeratorSource=Input port  DenominatorSource=Input port  ExternalReset=Rising  a0EqualsOne=on
      settings: InputPortMap=u0,p1,p3,r7
  Get_Current_Output_Offset : Subsystem
  Get_Current_delayed_Input_Offset : Subsystem
  NOT : Logic  Operator=NOT  IconShape=distinctive  AllPortsSameDT=off  OutDataTypeStr=boolean
  NOT1 : Logic  Operator=NOT  IconShape=distinctive  AllPortsSameDT=off  OutDataTypeStr=boolean
  Recursive Polynomial Model Estimator1 : slident/Estimators/Recursive Polynomial Model Estimator  ModelStructure=ARX  InitialEstimateSource=None  A0=2  B0=1  C0=1  D0=1  F0=1  nk=1  P0=10  InitialInputs=0  InitialOutputs=0  History=Infinite  WindowLength=2000  EstimationMethod=Forgetting Factor  AdaptationParameter=1  HasTimeVaryingAdaptationParameter=off  NormalizationBias=eps  OutputError=off  OutputP=off  AddEnablePort=on  ExternalReset=Rising  InputProcessing=Sample-based  Ts=1
      settings: SourceProductName=System Identification Toolbox  SourceProductBaseCode=ID
  Substract Current Offset so that the linearised model works : Sum  Inputs=+-
  Substract Current Offset so that the linearised model works1 : Sum  Inputs=+-
  System_Delay_Simulation : Delay  DelayLengthSource=Input port  DelayLength=600  DelayLengthUpperLimit=800  ExternalReset=Rising  SampleTime=1
      settings: InputPortMap=u0,p1,r5
  Vorsicht wenn resettet wird muss erst dieser Totzeitspeicher voll gelaufen sein bevor die Adaption starten darf Sonst kommt heir immer 0 raus und die Identifikation kann nicht rechnen : Constant  Value=0
  input Signal Low Pass Filter : DiscreteTransferFcn  Numerator=[0.01]  Denominator=[1 -0.99]  ExternalReset=Rising  SampleTime=1  a0EqualsOne=on
      settings: InputPortMap=u0,r7
  output Signal Low Pass Filter1 : DiscreteTransferFcn  Numerator=[0.01]  Denominator=[1 -0.99]  ExternalReset=Rising  SampleTime=1  a0EqualsOne=on
      settings: InputPortMap=u0,r7
  Gain_Filtered : Outport
  Gain_Not_Filtered : Outport  Port=2
  wires:
  Recursive Polynomial Model Estimator1/1 -> Bus Selector1/1
  input Signal Low Pass Filter/1 -> Recursive Polynomial Model Estimator1/1  "input"
  Bus Creator1/1 -> Calculate DC Gain1/1(Params)
  Bus Selector1/1 -> Bus Creator1/1  "<A>"
  Bus Selector1/2 -> Bus Creator1/2  "<B>"
  Substract Current Offset so that the linearised model works/1 -> output Signal Low Pass Filter1/1  "output minus mean"
  NOT/1 -> Get_Current_Output_Offset/Enable
  Get_Current_Output_Offset/1(Hold when disabled) -> Substract Current Offset so that the linearised model works/2
  System_Output/1 -> Get_Current_Output_Offset/1(In1), Substract Current Offset so that the linearised model works/1
  Get_Current_delayed_Input_Offset/1(Hold when disabled) -> Substract Current Offset so that the linearised model works1/2
  NOT1/1 -> Get_Current_delayed_Input_Offset/Enable
  Estimated Gain Tiefpassfilter/1 -> Gain_Filtered/1
  System_Input/1 -> System_Delay_Simulation/1  "real input"
  Vorsicht wenn resettet wird muss erst dieser Totzeitspeicher voll gelaufen sein bevor die Adaption starten darf Sonst kommt heir immer 0 raus und die Identifikation kann nicht rechnen/1 -> System_Delay_Simulation/3
  Dead_Time/1 -> System_Delay_Simulation/2
  Substract Current Offset so that the linearised model works1/1 -> input Signal Low Pass Filter/1  "imput delayed minus"
  System_Delay_Simulation/1 -> Substract Current Offset so that the linearised model works1/1, Get_Current_delayed_Input_Offset/1(In1)  "input delayed"
  Calculate DC Gain1/1(Calculated_Gain) -> Gain_Not_Filtered/1, Estimated Gain Tiefpassfilter/1
  Constant3/1 -> Estimated Gain Tiefpassfilter/2  "Num"
  Constant4/1 -> Estimated Gain Tiefpassfilter/3  "Den"
  Start_Identification/1 -> NOT/1, NOT1/1, Estimated Gain Tiefpassfilter/4, Recursive Polynomial Model Estimator1/4, output Signal Low Pass Filter1/2, input Signal Low Pass Filter/2, Recursive Polynomial Model Estimator1/3
  output Signal Low Pass Filter1/1 -> Recursive Polynomial Model Estimator1/2

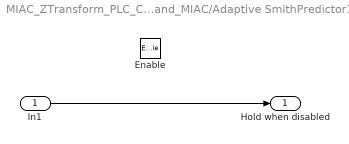
== system MIAC_ZTransform_PLC_Coder_not_external/Smith_Predictor_and_MIAC/Adaptive SmithPredictor1/Get_Current_Offset ==
  In1 : Inport
  Enable : EnablePort
  Hold when disabled : Outport
  wires:
  In1/1 -> Hold when disabled/1

== system MIAC_ZTransform_PLC_Coder_not_external/Smith_Predictor_and_MIAC/Adaptive SmithPredictor1/Get_Current_Offset1 ==
  In1 : Inport
  Enable : EnablePort
  Hold when disabled : Outport
  wires:
  In1/1 -> Hold when disabled/1

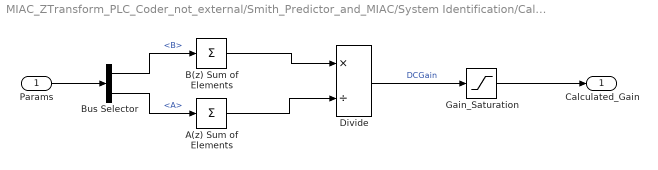
== system MIAC_ZTransform_PLC_Coder_not_external/Smith_Predictor_and_MIAC/System Identification/Calculate DC Gain1 ==
  Params : Inport
  A(z) Sum of Elements : Sum  Inputs=+
  B(z) Sum of Elements : Sum  Inputs=+
  Bus Selector : BusSelector  OutputSignals=B,A
  Divide : Product  Inputs=*/
  Gain_Saturation : Saturate  UpperLimit=1.5  LowerLimit=0.01
  Calculated_Gain : Outport
  wires:
  Params/1 -> Bus Selector/1
  Bus Selector/1 -> B(z) Sum of Elements/1  "<B>"
  Bus Selector/2 -> A(z) Sum of Elements/1  "<A>"
  B(z) Sum of Elements/1 -> Divide/1
  Divide/1 -> Gain_Saturation/1  "DCGain"
  A(z) Sum of Elements/1 -> Divide/2
  Gain_Saturation/1 -> Calculated_Gain/1

== system MIAC_ZTransform_PLC_Coder_not_external/Smith_Predictor_and_MIAC/System Identification/Get_Current_Output_Offset ==
  In1 : Inport
  Enable : EnablePort
  Hold when disabled : Outport
  wires:
  In1/1 -> Hold when disabled/1

== system MIAC_ZTransform_PLC_Coder_not_external/Smith_Predictor_and_MIAC/System Identification/Get_Current_delayed_Input_Offset ==
  In1 : Inport
  Enable : EnablePort
  Hold when disabled : Outport
  wires:
  In1/1 -> Hold when disabled/1

== system MIAC_ZTransform_PLC_Coder_not_external/Smith_Predictor_and_MIAC1/Adaptive SmithPredictor1/Get_Current_Offset ==
  In1 : Inport
  Enable : EnablePort
  Hold when disabled : Outport
  wires:
  In1/1 -> Hold when disabled/1

== system MIAC_ZTransform_PLC_Coder_not_external/Smith_Predictor_and_MIAC1/Adaptive SmithPredictor1/Get_Current_Offset1 ==
  In1 : Inport
  Enable : EnablePort
  Hold when disabled : Outport
  wires:
  In1/1 -> Hold when disabled/1

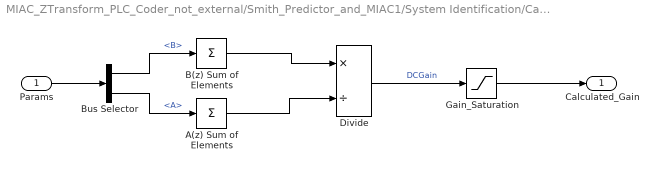
== system MIAC_ZTransform_PLC_Coder_not_external/Smith_Predictor_and_MIAC1/System Identification/Calculate DC Gain1 ==
  Params : Inport
  A(z) Sum of Elements : Sum  Inputs=+
  B(z) Sum of Elements : Sum  Inputs=+
  Bus Selector : BusSelector  OutputSignals=B,A
  Divide : Product  Inputs=*/
  Gain_Saturation : Saturate  UpperLimit=1.5  LowerLimit=0.01
  Calculated_Gain : Outport
  wires:
  Params/1 -> Bus Selector/1
  Bus Selector/1 -> B(z) Sum of Elements/1  "<B>"
  Bus Selector/2 -> A(z) Sum of Elements/1  "<A>"
  B(z) Sum of Elements/1 -> Divide/1
  Divide/1 -> Gain_Saturation/1  "DCGain"
  A(z) Sum of Elements/1 -> Divide/2
  Gain_Saturation/1 -> Calculated_Gain/1

== system MIAC_ZTransform_PLC_Coder_not_external/Smith_Predictor_and_MIAC1/System Identification/Get_Current_Output_Offset ==
  In1 : Inport
  Enable : EnablePort
  Hold when disabled : Outport
  wires:
  In1/1 -> Hold when disabled/1

== system MIAC_ZTransform_PLC_Coder_not_external/Smith_Predictor_and_MIAC1/System Identification/Get_Current_delayed_Input_Offset ==
  In1 : Inport
  Enable : EnablePort
  Hold when disabled : Outport
  wires:
  In1/1 -> Hold when disabled/1
